simulink model "roboTemplate"  (R2019a)
settings: Solver=ode23s  StartTime=tSim(1)  StopTime=tSim(end)  FixedStep=tStep  RelTol=1e-3  EnableMultiTasking=on
values from neighbouring files (symbols this model uses):
  dp = 0    [roboMain.m]
  ds = 7.2e-3    (= 0.0072)    [roboMain.m]
  g = 9.81    [berechnung.m]    (also in roboMain.m)
  IC = [phiStart, phi_dotStart, xStart x_dotStart]    [roboMain.m]
  l = 1    [berechnung.m]    (also in roboMain.m)
  L = 5    [berechnung.m]    (also in lagrange.m = T_pendel+T_schlitten-U_pendel; roboMain.m)
  ms = 0.8    [berechnung.m]    (also in roboMain.m)
  phi_max = pi/4    (= 0.785398163397)    [berechnung.m]    (also in roboMain.m)
  Pmax = wMmax*Mmax    (= 3.56)    [roboMain.m]
  r = 0.041    [berechnung.m]    (also in roboMain.m)
  Stoerung1 = .1    (= 0.1)    [roboMain.m]
  umax = 100    [roboMain.m]
libraries: simulink x1
settings Model: Creator=loehning  LastModifiedBy=Michael Hertneck
settings DataIOCC: SaveFormat=Array  SignalLoggingSaveFormat=ModelDataLogs  ReturnWorkspaceOutputs=off
settings OptimizationCC: ExpressionDepthLimit=2147483647  LifeSpan=inf
settings DebuggingCC: UnderspecifiedInitializationDetection=Classic  MergeDetectMultiDrivingBlocksExec=none  SolverPrmCheckMsg=warning  FcnCallInpInsideContextMsg=warning  StateNameClashWarn=warning  PregeneratedLibrarySubsystemCodeDiagnostic=none  SFUnexpectedBacktrackingDiag=warning  SFNoUnconditionalDefaultTransitionDiag=warning  SFExecutionAtInitializationDiag=none  ArithmeticOperatorsInVariantConditions=warning
settings HardwareCC: ProdBitPerPointer=32  ProdBitPerSizeT=32  ProdBitPerPtrDiffT=32  ProdLargestAtomicFloat=None  ProdIntDivRoundTo=Undefined  ProdEndianess=Unspecified  ProdWordSize=32  ProdHWDeviceType=32-bit Generic
settings ModelReferenceCC: PropagateSignalLabelsOutOfModel=off
settings SFSimCC: SimUseLocalCustomCode=off
settings RTWCC: RTWUseLocalCustomCode=off
settings CodeAppCC: StateflowObjectComments=on
settings GRTTargetCC: TargetLangStandard=C89/C90 (ANSI)  GeneratePreprocessorConditionals=Disable all  CombineOutputUpdateFcns=off  GRTInterface=on
settings ConfigComp: CovMetricSettings=dw  CovHtmlReporting=on  CovSaveCumulativeToWorkspaceVar=on  CovSaveSingleToWorkspaceVar=on  CovExternalEMLEnable=off  CovSFcnEnable=off

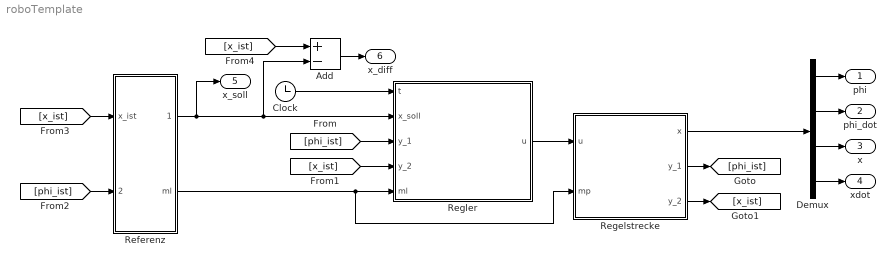
== system roboTemplate ==
  Add : Sum  Inputs=+-
  Clock : Clock
  Demux : Demux
  "Referenz " : Subsystem
  Regelstrecke : Subsystem
  Regler : Subsystem
  phi : Outport
  phi_dot : Outport  Port=2
  x : Outport  Port=3
  xdot : Outport  Port=4
  x_soll : Outport  Port=5
  x_diff : Outport  Port=6
  wires:
  [phi_ist] -> Regler/3(y_1)
  Regelstrecke/1(x) -> Demux/1
  [x_ist] -> Add/1
  [x_ist] -> Regler/4(y_2)
  [x_ist] -> "Referenz "/1(x_ist)
  Demux/3 -> x/1
  Regelstrecke/3(y_2) -> [x_ist]
  Regelstrecke/2(y_1) -> [phi_ist]
  [phi_ist] -> "Referenz "/2(phi_ist)
  Demux/2 -> phi_dot/1
  "Referenz "/1("x_soll ") -> Regler/2("x_soll "), Add/2, x_soll/1
  Regler/1(u) -> Regelstrecke/1("u ")
  Demux/1 -> phi/1
  Demux/4 -> xdot/1
  Add/1 -> x_diff/1
  "Referenz "/2(ml) -> Regler/5(ml), Regelstrecke/2(mp)
  Clock/1 -> Regler/1(t)

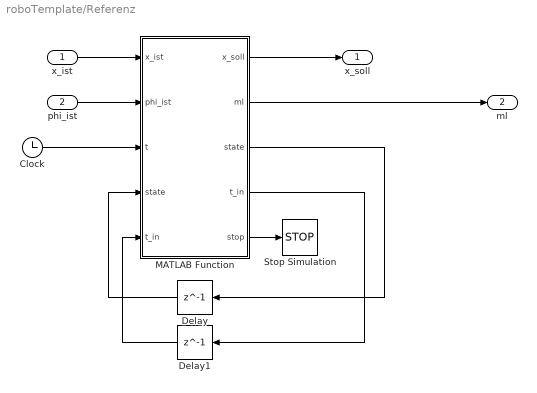
== system roboTemplate/Referenz  ==
  x_ist : Inport
  phi_ist : Inport  Port=2
  Clock : Clock
  Delay : Delay  DelayLength=1  InitialCondition=1  SampleTime=0.025
  Delay1 : Delay  DelayLength=1  SampleTime=0.025
  MATLAB Function : MATLAB Function  TreatAsAtomicUnit=on
  Stop Simulation : Stop
  "x_soll " : Outport
  ml : Outport  Port=2
  wires:
  MATLAB Function/3(state) -> Delay/1
  Delay/1 -> MATLAB Function/4("state ")
  Clock/1 -> MATLAB Function/3(t)
  x_ist/1 -> MATLAB Function/1(x_ist)
  phi_ist/1 -> MATLAB Function/2(phi_ist)
  MATLAB Function/1(x_soll) -> "x_soll "/1
  MATLAB Function/4(t_in) -> Delay1/1
  Delay1/1 -> MATLAB Function/5("t_in ")
  MATLAB Function/5(stop) -> Stop Simulation/1
  MATLAB Function/2(ml) -> ml/1

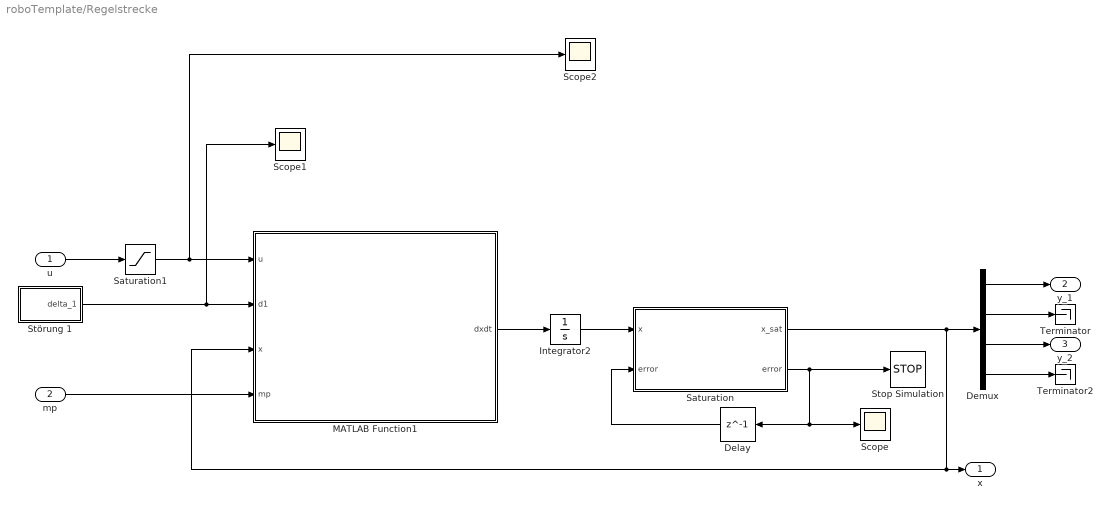
== system roboTemplate/Regelstrecke ==
  "u " : Inport
  mp : Inport  Port=2
  Delay : Delay  DelayLength=1  InitialCondition=0  SampleTime=0.025
  Demux : Demux
  Integrator2 : Integrator  InitialCondition=IC
  MATLAB Function1 : MATLAB Function  TreatAsAtomicUnit=on
  "Saturation " : MATLAB Function  TreatAsAtomicUnit=on
  Saturation1 : Saturate  UpperLimit=umax  LowerLimit=-umax
  Scope : Scope
  Scope1 : Scope
  Scope2 : Scope
  Stop Simulation : Stop
  Störung 1 : Subsystem
  Terminator : Terminator
  Terminator2 : Terminator
  x : Outport
  y_1 : Outport  Port=2
  y_2 : Outport  Port=3
  wires:
  MATLAB Function1/1(dxdt) -> Integrator2/1
  "Saturation "/1(x_sat) -> Demux/1, MATLAB Function1/3(x), x/1
  "u "/1 -> Saturation1/1
  Saturation1/1 -> MATLAB Function1/1(u), Scope2/1
  mp/1 -> MATLAB Function1/4(mp)
  Delay/1 -> "Saturation "/2("error ")
  Demux/1 -> y_1/1
  Demux/3 -> y_2/1
  Demux/4 -> Terminator2/1
  Demux/2 -> Terminator/1
  Integrator2/1 -> "Saturation "/1(x)
  "Saturation "/2(error) -> Stop Simulation/1, Delay/1, Scope/1
  Störung 1/1("delta_1 ") -> MATLAB Function1/2(d1), Scope1/1

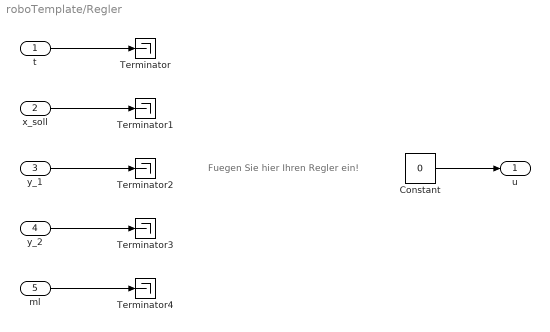
== system roboTemplate/Regler ==
  note: Fuegen Sie hier Ihren Regler ein!
  t : Inport
  "x_soll " : Inport  Port=2
  y_1 : Inport  Port=3
  y_2 : Inport  Port=4
  ml : Inport  Port=5
  Constant : Constant  Value=0
  Terminator{,1..4} (5 alike) : Terminator
  u : Outport
  wires:
  t/1 -> Terminator/1
  "x_soll "/1 -> Terminator1/1
  y_1/1 -> Terminator2/1
  y_2/1 -> Terminator3/1
  ml/1 -> Terminator4/1
  Constant/1 -> u/1

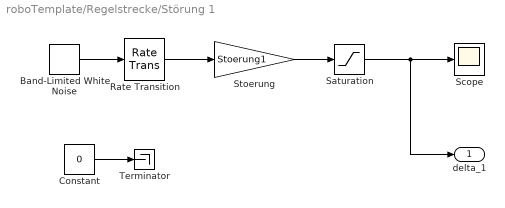
== system roboTemplate/Regelstrecke/Störung 1 ==
  Band-Limited White Noise : simulink/Sources/Band-Limited White Noise  Cov=stoerungNoisePower  Ts=0.025  seed=stoerungSeed_1
  Constant : Constant  Value=0
  Rate Transition : RateTransition
  Saturation : Saturate  UpperLimit=3  LowerLimit=-3
  Scope : Scope
  Stoerung : Gain  Gain=Stoerung1
  Terminator : Terminator
  "delta_1 " : Outport
  wires:
  Band-Limited White Noise/1 -> Rate Transition/1
  Rate Transition/1 -> Stoerung/1
  Stoerung/1 -> Saturation/1
  Saturation/1 -> "delta_1 "/1, Scope/1
  Constant/1 -> Terminator/1

== matlab function roboTemplate/Referenz /MATLAB Function ==
  data: x_ist input; x_soll output; ml output; phi_ist input; t input; state input; state output; t_in input; t_in output; stop output
%Dies ist ein Beispiel fuer die Referenzfunktion. Die Referenzpunkte können
%veraendert werden, indem Eintraege in x_ref_vec ergaenzt oder entfernt
%werden. Entsprechend muss in ml_vec jeweils ein Wert für m_l zu jedem
%Referenzpunkt gewaehlt werden. 
%!Beachten Sie dass fuer die Wettberwebsaufgabe andere Referenzpunkte und
%Massen gewaehlt werden!.

function [x_soll,ml,state,t_in,stop] = reference(x_ist,phi_ist,t,state,t_in)
%x_bound und phi_bound geben eine Umgebung um den jeweiligen Referenzpunkt
%und um phi = 0 vor, in der der Regler das System für die Zeit t_bound
%trotz der Stoerung halten muss, damit der Referenzpunkt als erreicht
%betrachtet wird.
x_bound = 2*10^-2;
phi_bound = 2*10^-2;
t_bound = 1.5;
stop = 0;

%Hier können Referenzpunkte gewählt werden.
x_ref_vec = [0.2,-2,2,-2.45,1,1.1,1.2,2,0];
ml_vec = [1,3,2,1,5,1,4,2,5];

if(state <= size(x_ref_vec,2))
    x_soll = x_ref_vec(state);
    ml = ml_vec(state);
    if(abs(x_ist-x_ref_vec(state)) > x_bound)
        t_in = t;
    end
    if(abs(phi_ist-0) > phi_bound)
        t_in = t;
    end
    if(t-t_in > t_bound)
        state = state+1;
        t_in = t;
    end
    
else
    x_soll = x_ref_vec(size(x_ref_vec,2));
    ml = ml_vec(size(x_ref_vec,2));
    stop = 1;
end

== matlab function roboTemplate/Regelstrecke/Saturation  ==
  data: x input size=[1,4]; error input; phi_max parameter; x_sat output size=[1,4]; L parameter; error output
function [x_sat,error]  = fcn(x, error,phi_max, L)


x_sat = x;

%Saturation in x
if x(3) >= L/2
    x_sat(3) = L/2;
    x_sat(4) = 0; %Roboter fällt herunter!!!!
    error = 1;
end

if x(3) <= -L/2
    x_sat(3) = -L/2;
    x_sat(4) = 0; %Roboter fällt herunter!!!!
    error = 1;
end

%Saturation in phi
if (abs(x(1)) > phi_max) 
    error = 1;
end

if (error)
    x_sat = zeros(1,4);
end

== matlab function roboTemplate/Regelstrecke/MATLAB Function1 ==
  data: u input; d1 input; dxdt output size=[1 4]; x input size=[1 4]; g parameter; ms parameter; l parameter; Pmax parameter; umax parameter; r parameter; ds parameter; dp parameter; mp input
function dxdt   = dynamikStrecke(u, d1, x, g, ms, l, Pmax, umax, r,ds,dp, mp)


%Berechnung des Motormomentes
P = (u+d1)/umax*Pmax; %Leistung eines Motors
M_max = sqrt(abs(P))/9.434;

M = 2*sign2(u+d1)*M_max; % Gesamtmoment


%Systemdynamik
phi = x(1);
dphi = x(2);
w = x(3);
dw = x(4);

dxdt = zeros(1,4);  
dxdt = statespace_model(M,g, ms, l, r,ds,dp, mp,w,dw,phi,dphi,x); %Hier wird direkt die Lösung zu Aufgabe 4.2.1 verwendet. Um diese nicht direkt zu verraten ist sie in der geschützten Funktion statespace_model.p implementiert.


end
function u =  sign2(x)
    if(x == 0) 
        u = -1;
    else
        u = sign(x);
    end
end
